simulink model "adaptive_dcmotor_sim"  (R2025b)
settings: Solver=FixedStepDiscrete  StartTime=0.0  StopTime=96  FixedStep=0.08  RelTol=1e-3
settings Model: Creator=Lenard  LastModifiedBy=Lenard

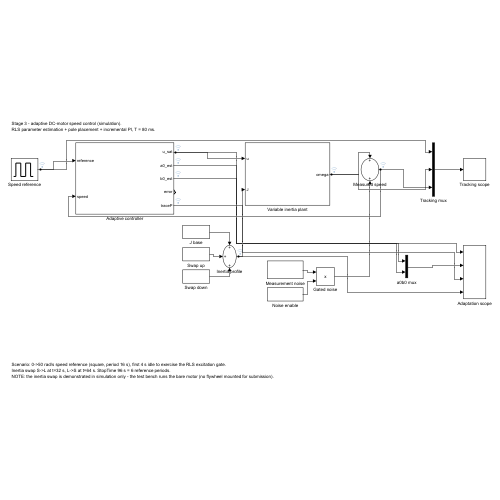
[thumbnail: Simulink's stored preview of the top-level diagram]
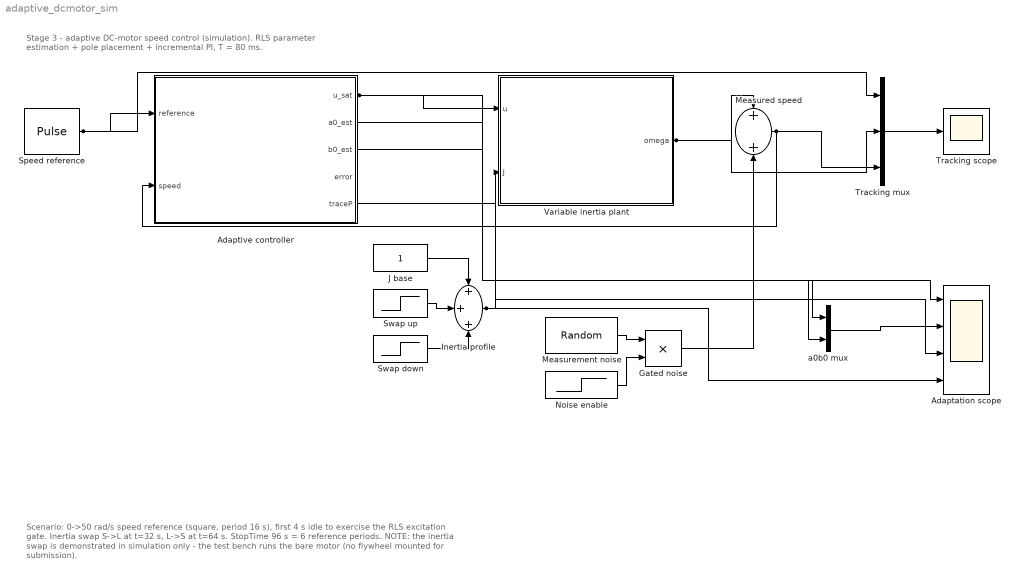
== system adaptive_dcmotor_sim ==
  note: Stage 3 - adaptive DC-motor speed control (simulation).
      | RLS parameter estimation + pole placement + incremental PI, T = 80 ms.
  note: Scenario: 0->50 rad/s speed reference (square, period 16 s), first 4 s idle to exercise the RLS excitation gate.
      | Inertia swap S->L at t=32 s, L->S at t=64 s. StopTime 96 s = 6 reference periods.
      | NOTE: the inertia swap is demonstrated in simulation only - the test bench runs the bare motor (no flywheel mounted for submission).
  Adaptation scope : Scope  NumInputPorts=4
  Adaptive controller : Subsystem
  Gated noise : Product
  Inertia profile : Sum  Inputs=+++
  J base : Constant
  Measured speed : Sum
  Measurement noise : RandomNumber  Variance=0.0125  Seed=23341  SampleTime=0.08
  Noise enable : Step  Time=4  SampleTime=0.08
  Speed reference : DiscretePulseGenerator  PulseType=Time based  Amplitude=50  Period=16  PulseWidth=50  PhaseDelay=4  SampleTime=0.08
  Swap down : Step  Time=64  After=-23  SampleTime=0.08
  Swap up : Step  Time=32  After=23  SampleTime=0.08
  Tracking mux : Mux  Inputs=3
  Tracking scope : Scope
  Variable inertia plant : Subsystem
  a0b0 mux : Mux  Inputs=2
  wires:
  Speed reference/1 -> Adaptive controller/1(reference), Tracking mux/1
  Adaptive controller/1(u_sat) -> Variable inertia plant/1(u), Adaptation scope/1
  J base/1 -> Inertia profile/1
  Swap up/1 -> Inertia profile/2
  Swap down/1 -> Inertia profile/3
  Inertia profile/1 -> Variable inertia plant/2(J), Adaptation scope/4
  Variable inertia plant/1(omega) -> Measured speed/1, Tracking mux/2
  Measurement noise/1 -> Gated noise/1
  Noise enable/1 -> Gated noise/2
  Gated noise/1 -> Measured speed/2
  Measured speed/1 -> Adaptive controller/2(speed), Tracking mux/3
  Tracking mux/1 -> Tracking scope/1
  Adaptive controller/2(a0_est) -> a0b0 mux/1
  Adaptive controller/3(b0_est) -> a0b0 mux/2
  a0b0 mux/1 -> Adaptation scope/2
  Adaptive controller/5(traceP) -> Adaptation scope/3

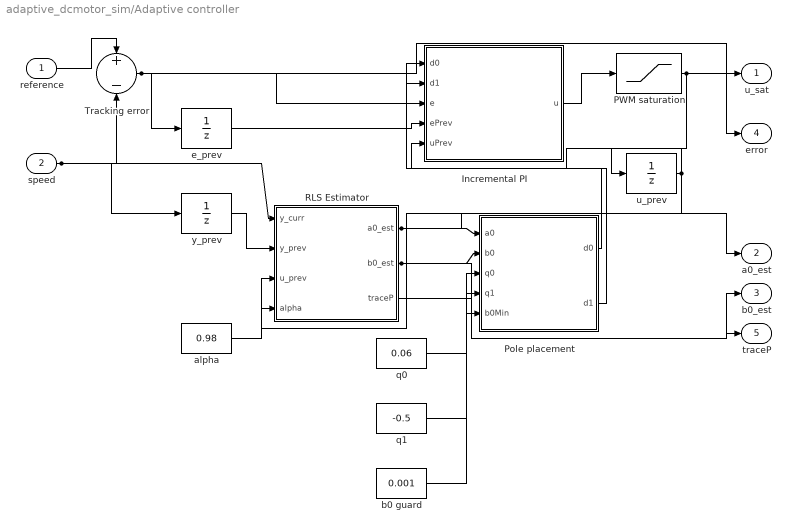
== system adaptive_dcmotor_sim/Adaptive controller ==
  reference : Inport
  speed : Inport  Port=2
  Incremental PI : MATLAB Function  TreatAsAtomicUnit=on
  PWM saturation : Saturate  UpperLimit=255  LowerLimit=-255
  Pole placement : MATLAB Function  TreatAsAtomicUnit=on
  RLS Estimator : MATLAB Function  TreatAsAtomicUnit=on
  Tracking error : Sum  Inputs=+-
  alpha : Constant  Value=0.98
  b0 guard : Constant  Value=0.001
  e_prev : UnitDelay  SampleTime=0.08  HasFrameUpgradeWarning=on
  q0 : Constant  Value=0.06
  q1 : Constant  Value=-0.5
  u_prev : UnitDelay  SampleTime=0.08  HasFrameUpgradeWarning=on
  y_prev : UnitDelay  SampleTime=0.08  HasFrameUpgradeWarning=on
  u_sat : Outport
  a0_est : Outport  Port=2
  b0_est : Outport  Port=3
  error : Outport  Port=4
  traceP : Outport  Port=5
  wires:
  reference/1 -> Tracking error/1
  speed/1 -> Tracking error/2, y_prev/1, RLS Estimator/1(y_curr)
  Tracking error/1 -> e_prev/1, Incremental PI/3(e), error/1
  y_prev/1 -> RLS Estimator/2(y_prev)
  u_prev/1 -> RLS Estimator/3(u_prev), Incremental PI/5(uPrev)
  alpha/1 -> RLS Estimator/4(alpha)
  RLS Estimator/1(a0_est) -> Pole placement/1(a0), a0_est/1
  RLS Estimator/2(b0_est) -> Pole placement/2(b0), b0_est/1
  RLS Estimator/3(traceP) -> traceP/1
  q0/1 -> Pole placement/3(q0)
  q1/1 -> Pole placement/4(q1)
  b0 guard/1 -> Pole placement/5(b0Min)
  Pole placement/1(d0) -> Incremental PI/1(d0)
  Pole placement/2(d1) -> Incremental PI/2(d1)
  e_prev/1 -> Incremental PI/4(ePrev)
  Incremental PI/1(u) -> PWM saturation/1
  PWM saturation/1 -> u_prev/1, u_sat/1

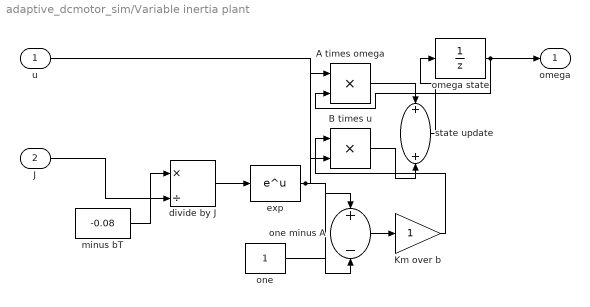
== system adaptive_dcmotor_sim/Variable inertia plant ==
  u : Inport
  J : Inport  Port=2
  A times omega : Product
  B times u : Product
  Km over b : Gain
  divide by J : Product  Inputs=*/
  exp : Math
  minus bT : Constant  Value=-0.08
  omega state : UnitDelay  SampleTime=0.08  HasFrameUpgradeWarning=on
  one : Constant
  one minus A : Sum  Inputs=+-
  state update : Sum
  omega : Outport
  wires:
  J/1 -> divide by J/2
  minus bT/1 -> divide by J/1
  divide by J/1 -> exp/1
  exp/1 -> one minus A/2, A times omega/1
  one/1 -> one minus A/1
  one minus A/1 -> Km over b/1
  omega state/1 -> A times omega/2, omega/1
  Km over b/1 -> B times u/1
  u/1 -> B times u/2
  A times omega/1 -> state update/1
  B times u/1 -> state update/2
  state update/1 -> omega state/1

== matlab function adaptive_dcmotor_sim/Adaptive controller/Pole placement ==
  data: a0 input; d0 output; b0 input; q0 input; q1 input; b0Min input; d1 output
function [d0,d1] = pole_placement(a0,b0,q0,q1,b0Min)            
                                                               %#codegen                                                       
                                                               % Hold the previous gains while |b0| is too small (guard against
                                                               % division blow-up before the estimator has converged).         
                                                               persistent d0Hold d1Hold                                        
                                                               if isempty(d0Hold)                                              
                                                                   d0Hold = -0.44;                                             
                                                                   d1Hold = 1.0;                                               
                                                               end                                                             
                                                               if abs(b0) > b0Min                                              
                                                                   d0Hold = (q0 + a0) / b0;                                    
                                                                   d1Hold = (q1 + 1.0 - a0) / b0;                              
                                                               end                                                             
                                                               d0 = d0Hold;                                                    
                                                               d1 = d1Hold;                                                    
                                                               end

== matlab function adaptive_dcmotor_sim/Adaptive controller/RLS Estimator ==
  data: y_curr input; a0_est output; y_prev input; u_prev input; alpha input; b0_est output; traceP output
function [a0_est,b0_est,traceP] = rls_estimator(y_curr,y_prev,u_prev,alpha)
                                                                          %#codegen                                                                  
                                                                          % RLS for G(z) = b0/(z + a0). Excitation gate: skip the update when        
                                                                          % the regressor is ~zero (motor idle) so P = P/alpha cannot wind up.       
                                                                          persistent P xe                                                            
                                                                          if isempty(P)                                                              
                                                                              P = 100.0 * eye(2);                                                    
                                                                              xe = [-0.5; 1.0];                                                      
                                                                          end                                                                        
                                                                          C = [-y_prev, u_prev];                                                     
                                                                          if (C * C') > 1e-6                                                         
                                                                              den = C * P * C' + alpha;                                              
                                                                              L = (P * C') / den;                                                    
                                                                              xe = xe + L * (y_curr - C * xe);                                       
                                                                              P = (eye(2) - L * C) * P / alpha;                                      
                                                                              P = 0.5 * (P + P');                                                    
                                                                          end                                                                        
                                                                          a0_est = xe(1);                                                            
                                                                          b0_est = xe(2);                                                            
                                                                          traceP = P(1,1) + P(2,2);                                                  
                                                                          end

== matlab function adaptive_dcmotor_sim/Adaptive controller/Incremental PI ==
  data: d0 input; u output; d1 input; e input; ePrev input; uPrev input
function u = incremental_pi(d0,d1,e,ePrev,uPrev)
                                               %#codegen                                       
                                               u = uPrev + d1 * e + d0 * ePrev;                
                                               end
